simulink model "zad_5_sch_ciagly"  (R2022b)
settings: Solver=FixedStepAuto  StartTime=0.0  StopTime=5  FixedStep=0.001  RelTol=1e-3
values from neighbouring files (symbols this model uses):
  a21 = 1/(2*m)*x30^2*FemP1/FemP2^2*exp(-x10/FemP2)    [zad_5.m]
  a23 = -1/(m)*x30*FemP1/FemP2*exp(-x10/FemP2)    [zad_5.m]
  a31 = 1/f1*exp(x10/f2)*(ki*u10+ci-x30)    [zad_5.m]
  a33 = -f2/f1*exp(x10/f2)    [zad_5.m]
  b31 = ki*f2/f1*exp(x10/f2)    [zad_5.m]
  g = 9.81    [zad_5.m]
  Kx = -acker(A, B(:,1), -sKx)    [zad_5.m]
  Lo = acker(A', C', -sLo)    [zad_5.m]
  u0 = -(a31*x1+a33*x3)/b31    [zad_5.m]
  u10 = 1/ki*(x30-ci)    [zad_5.m]
  x1 = .003    (= 0.003)    [zad_5.m]
  x2 = 0    [zad_5.m]
  x3 = -(a21*x1+g)/a23    [zad_5.m]
  xd = d-bd    (= 0.0192)    [zad_5.m]
settings Model: Creator=AgraWoodAdmin  LastModifiedBy=AgraWoodAdmin
settings DebuggingCC: UnconnectedInputMsg=warning  UnconnectedOutputMsg=warning  UnconnectedLineMsg=warning
settings ModelReferenceCC: EnableRefExpFcnMdlSchedulingChecks=on
settings RTWCC: DLArmComputeVersion=19.05

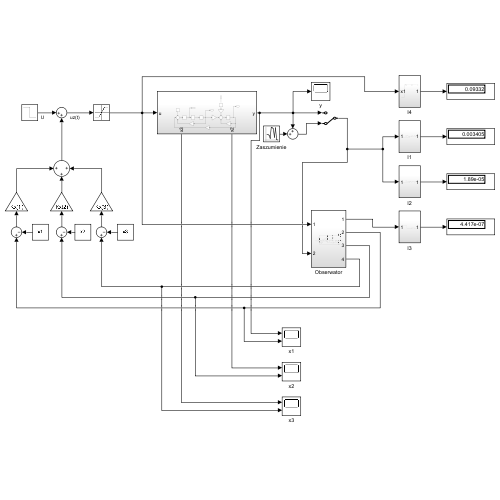
[thumbnail: Simulink's stored preview of the top-level diagram]
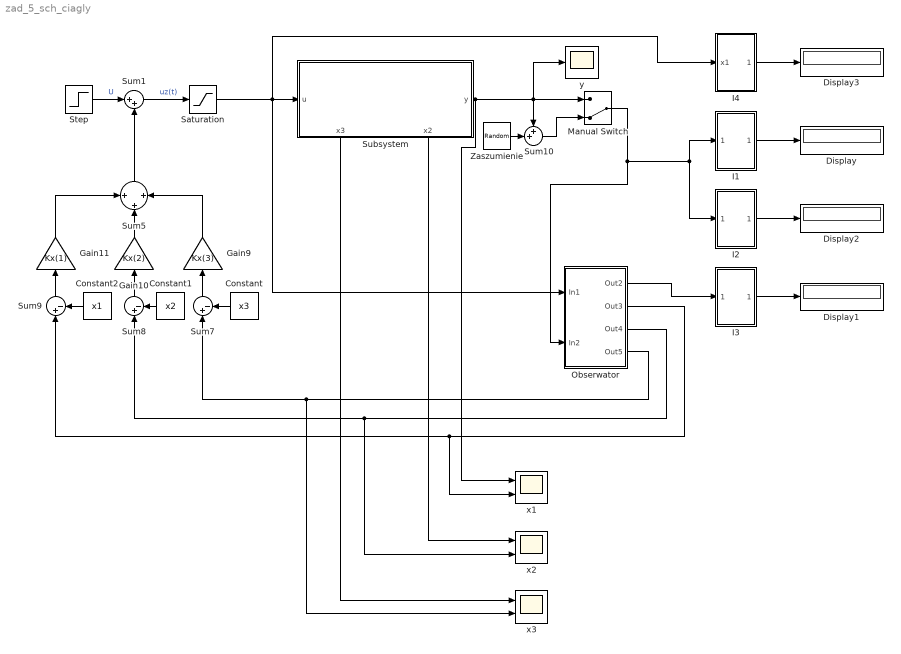
== system zad_5_sch_ciagly ==
  Constant : Constant  Value=x3
  Constant1 : Constant  Value=x2
  Constant2 : Constant  Value=x1
  Display{,1..3} (4 alike) : Display
  Gain10 : Gain  Gain=Kx(2)
  Gain11 : Gain  Gain=Kx(1)
  Gain9 : Gain  Gain=Kx(3)
  I1 : Subsystem
  I2 : Subsystem
  I3 : Subsystem
  I4 : Subsystem
  Manual Switch : ManualSwitch  CurrentSetting=0
  Obserwator : Subsystem
  Saturation : Saturate  UpperLimit=1  LowerLimit=0
  Step : Step  Time=0  Before=u10  After=u0  SampleTime=0
  Subsystem : Subsystem
      settings: PortSchema="{\"entries\":[{\"content\":{\"sides\":[{\"content\":{\"connectorIds\":[\"In1\"]},\"type\":\"ConnectorPlacement.EquallySpacedRectSide\",\"uuid\":\"a9618e66-a868-4602-adbc-d46c199391e9\"},{\"content\":{\"connectorIds\":[\"Out1\"],\"side\":\"RIGHT\"},\"type\":\"ConnectorPlacement.EquallySpacedRectSide\",\"uuid\":\"c3196c58-25c5-4c17-9484-b8d421343e51\"},{\"content\":{\"connectorIds\":[],\"side\":\"TOP\"},\"type\":\"ConnectorPlacement.EquallySpacedRectSide\",\"uuid\":\"906d255b-3a1d-4e09-a9da-ed665958d266\"},{\"content\":{\"connectorIds\":[\"Out2\",\"Out3\"],\"side\":\"BOTTOM\"},\"type\":\"ConnectorPlacement.EquallySpacedRectSide\",\"uuid\":\"d9e5422d-f936-4847-a7ac-e53a1bad6272\"}]},\"type\":\"ConnectorPlacement.EquallySpacedConnector\",\"uuid\":\"1b3fe789-ebdd-4120-9cfb-1ec5ed381a45\"}],\"packageUris\":[\"http://schema.mathworks.com/mf0/Connector/R2020b\"],\"version\":\"1.0\"}"
  Sum1 : Sum  Inputs=|++
  Sum10 : Sum  Inputs=++|
  Sum5 : Sum  Inputs=+|+|+
  Sum7 : Sum  Inputs=|+-
  Sum8 : Sum  Inputs=|+-
  Sum9 : Sum  Inputs=|+-
  Zaszumienie : RandomNumber  Variance=.0000001
  x1 : Scope  NumInputPorts=2
  x2 : Scope  NumInputPorts=2
  x3 : Scope  NumInputPorts=2
  y : Scope
  wires:
  Step/1 -> Sum1/1  "U"
  Subsystem/1(y) -> x1/1, y/1, Sum10/1, Manual Switch/1
  Sum1/1 -> Saturation/1  "uz(t)"
  Sum5/1 -> Sum1/2
  Constant/1 -> Sum7/2
  Sum7/1 -> Gain9/1
  Constant1/1 -> Sum8/2
  Sum8/1 -> Gain10/1
  Constant2/1 -> Sum9/2
  Sum9/1 -> Gain11/1
  Gain9/1 -> Sum5/3
  Gain10/1 -> Sum5/2
  Gain11/1 -> Sum5/1
  Manual Switch/1 -> I2/1(In1), I1/1(In1), Obserwator/2(In2)
  Sum10/1 -> Manual Switch/2
  I1/1(Out1) -> Display/1
  I3/1(Out1) -> Display1/1
  I2/1(Out1) -> Display2/1
  I4/1(Out1) -> Display3/1
  Saturation/1 -> Obserwator/1(In1), I4/1(x1), Subsystem/1(u)
  Obserwator/1(Out2) -> I3/1(In1)
  Obserwator/2(Out3) -> x1/2, Sum9/1
  Obserwator/3(Out4) -> x2/2, Sum8/1
  Obserwator/4(Out5) -> x3/2, Sum7/1
  Zaszumienie/1 -> Sum10/2
  Subsystem/3(x2) -> x2/1
  Subsystem/2(x3) -> x3/1

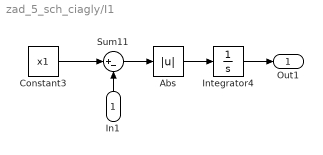
== system zad_5_sch_ciagly/I1 ==
  In1 : Inport
  Abs : Abs  SaturateOnIntegerOverflow=off
  Constant3 : Constant  Value=x1
  Integrator4 : Integrator
  Sum11 : Sum  Inputs=|+-
  Out1 : Outport
  wires:
  Constant3/1 -> Sum11/1
  Integrator4/1 -> Out1/1
  Sum11/1 -> Abs/1
  Abs/1 -> Integrator4/1
  In1/1 -> Sum11/2

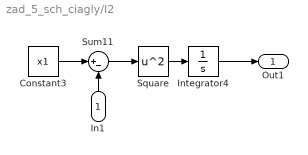
== system zad_5_sch_ciagly/I2 ==
  In1 : Inport
  Constant3 : Constant  Value=x1
  Integrator4 : Integrator
  Square : Math  Operator=square
  Sum11 : Sum  Inputs=|+-
  Out1 : Outport
  wires:
  Constant3/1 -> Sum11/1
  Integrator4/1 -> Out1/1
  Sum11/1 -> Square/1
  Square/1 -> Integrator4/1
  In1/1 -> Sum11/2

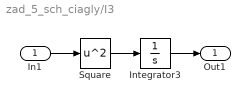
== system zad_5_sch_ciagly/I3 ==
  In1 : Inport
  Integrator3 : Integrator
  Square : Math  Operator=square
  Out1 : Outport
  wires:
  In1/1 -> Square/1
  Square/1 -> Integrator3/1
  Integrator3/1 -> Out1/1

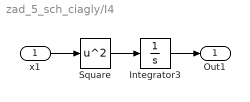
== system zad_5_sch_ciagly/I4 ==
  x1 : Inport
  Integrator3 : Integrator
  Square : Math  Operator=square
  Out1 : Outport
  wires:
  Integrator3/1 -> Out1/1
  Square/1 -> Integrator3/1
  x1/1 -> Square/1

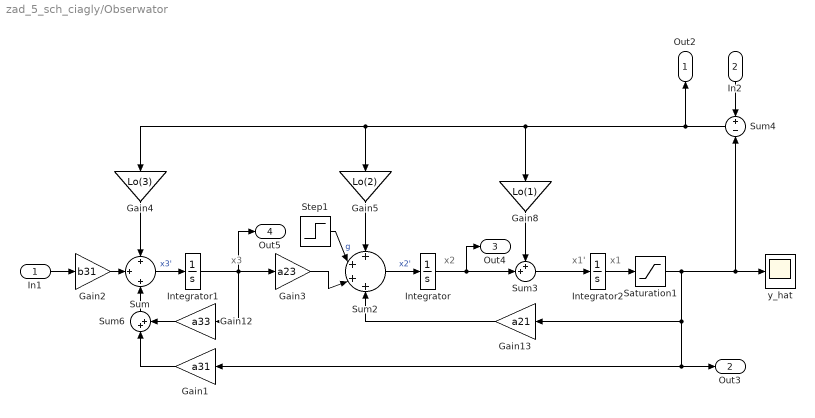
== system zad_5_sch_ciagly/Obserwator ==
  note: x3
  note: x1'
  note: x1
  note: x2
  In1 : Inport
  In2 : Inport  Port=2
  Gain1 : Gain  Gain=a31
  Gain12 : Gain  Gain=a33
  Gain13 : Gain  Gain=a21
  Gain2 : Gain  Gain=b31
  Gain3 : Gain  Gain=a23
  Gain4 : Gain  Gain=Lo(3)
  Gain5 : Gain  Gain=Lo(2)
  Gain8 : Gain  Gain=Lo(1)
  Integrator : Integrator
  Integrator1 : Integrator
  Integrator2 : Integrator  InitialCondition=xd
  Saturation1 : Saturate  UpperLimit=xd  LowerLimit=0
  Step1 : Step  Time=0  After=g  SampleTime=0
  Sum : Sum  Inputs=+|+|+
  Sum2 : Sum  Inputs=+|+|+|+
  Sum3 : Sum  Inputs=++|
  Sum4 : Sum  Inputs=+|-
  Sum6 : Sum  Inputs=|++
  y_hat : Scope
  Out2 : Outport
  Out3 : Outport  Port=2
  Out4 : Outport  Port=3
  Out5 : Outport  Port=4
  wires:
  Sum4/1 -> Gain4/1, Gain5/1, Gain8/1, Out2/1
  Saturation1/1 -> y_hat/1, Sum4/2, Out3/1, Gain1/1, Gain13/1
  Gain1/1 -> Sum6/1
  Step1/1 -> Sum2/2  "g"
  Gain8/1 -> Sum3/1
  Gain2/1 -> Sum/2
  Integrator1/1 -> Out5/1, Gain3/1, Gain12/1
  Gain4/1 -> Sum/1
  Gain5/1 -> Sum2/1
  Gain3/1 -> Sum2/3
  Sum6/1 -> Sum/3
  Integrator2/1 -> Saturation1/1
  In1/1 -> Gain2/1
  Gain13/1 -> Sum2/4
  Sum3/1 -> Integrator2/1
  Integrator/1 -> Out4/1, Sum3/2
  Gain12/1 -> Sum6/2
  Sum2/1 -> Integrator/1  "x2'"
  Sum/1 -> Integrator1/1  "x3'"
  In2/1 -> Sum4/1

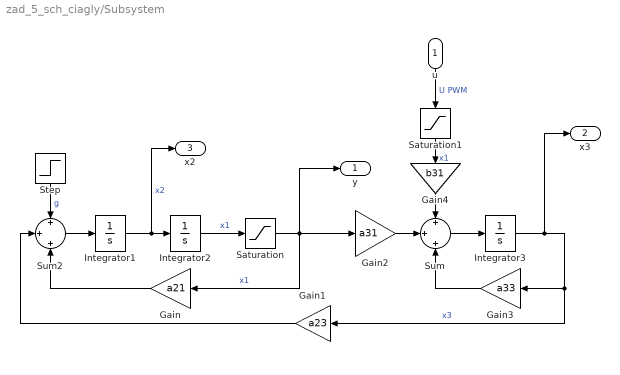
== system zad_5_sch_ciagly/Subsystem ==
  u : Inport
  Gain : Gain  Gain=a21
  Gain1 : Gain  Gain=a23
  Gain2 : Gain  Gain=a31
  Gain3 : Gain  Gain=a33
  Gain4 : Gain  Gain=b31
  Integrator1 : Integrator
  Integrator2 : Integrator  InitialCondition=xd
  Integrator3 : Integrator
  Saturation : Saturate  UpperLimit=xd  LowerLimit=0
  Saturation1 : Saturate  UpperLimit=1  LowerLimit=0
  Step : Step  Time=0  After=g  SampleTime=0
  Sum : Sum  Inputs=+|+|+
  Sum2 : Sum  Inputs=+|+|+
  y : Outport
  x3 : Outport  Port=2
  x2 : Outport  Port=3
  wires:
  Step/1 -> Sum2/1  "g"
  Integrator1/1 -> x2/1, Integrator2/1  "x2"
  Gain1/1 -> Sum2/2
  u/1 -> Saturation1/1  "U PWM"
  Saturation/1 -> Gain/1, Gain2/1, y/1  "x1"
  Integrator3/1 -> x3/1, Gain1/1, Gain3/1  "x3"
  Gain/1 -> Sum2/3
  Gain2/1 -> Sum/2
  Gain3/1 -> Sum/3
  Sum2/1 -> Integrator1/1
  Sum/1 -> Integrator3/1
  Integrator2/1 -> Saturation/1  "x1"
  Gain4/1 -> Sum/1
  Saturation1/1 -> Gain4/1  "x1"
